simulink model "tank_phase1"  (R2025b)
settings: Solver=ode45  StartTime=0.0  StopTime=900  RelTol=1e-3
model workspace (MAT data in the model file):
  pumpProfile = timeseries
  pumpProfile.Name = 'unnamed'
  pumpProfile.DataInfo = tsdata.datametadata
  pumpProfile.DataInfo.Interpolation = tsdata.interpolation
  pumpProfile.DataInfo.Interpolation.Fhandle : function handle (value not decoded)
  pumpProfile.DataInfo.Interpolation.Name = 'linear'
  pumpProfile.TimeInfo = tsdata.timemetadata
  pumpProfile.TimeInfo.Length = 3
  pumpProfile.TimeInfo.DuplicateTimes = 0
  pumpProfile.TimeInfo.Time_ = [0; 300; 600]
  pumpProfile.TimeInfo.Initialized = 1
  pumpProfile.QualityInfo = tsdata.qualmetadata
  pumpProfile.Data_ = [20; 40; 60]
settings Model: Creator=maild  LastModifiedBy=maild

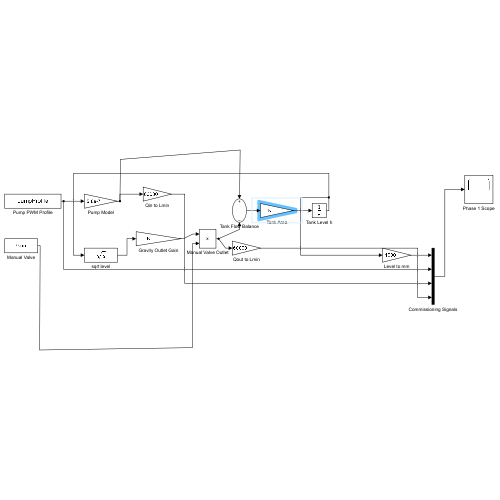
[thumbnail: Simulink's stored preview of the top-level diagram]
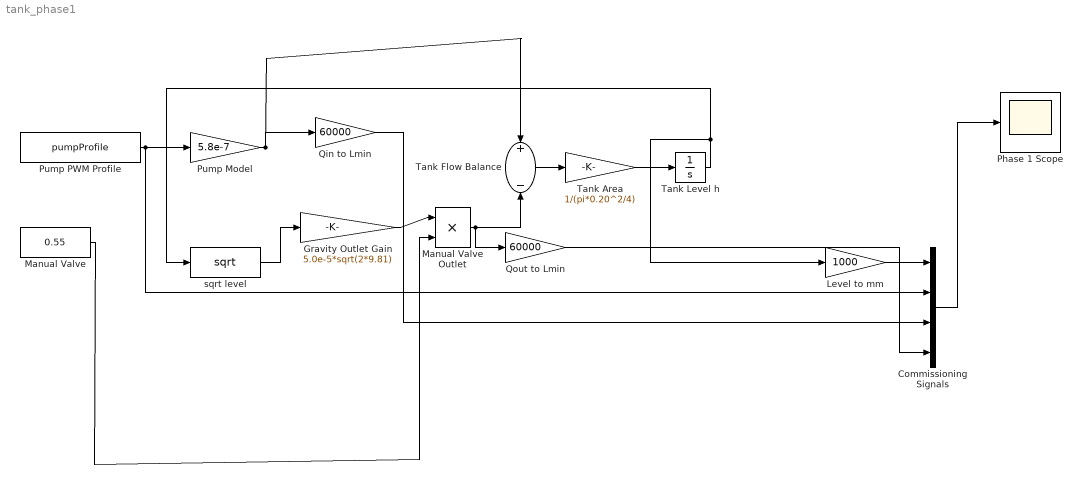
== system tank_phase1 ==
  Commissioning Signals : Mux
  Gravity Outlet Gain : Gain  Gain=5.0e-5*sqrt(2*9.81)
  Level to mm : Gain  Gain=1000
  Manual Valve : Constant  Value=0.55
  Manual Valve Outlet : Product
  Phase 1 Scope : Scope
  Pump Model : Gain  Gain=5.8e-7
  Pump PWM Profile : FromWorkspace  VariableName=pumpProfile
  Qin to Lmin : Gain  Gain=60000
  Qout to Lmin : Gain  Gain=60000
  Tank Area : Gain  Gain=1/(pi*0.20^2/4)
  Tank Flow Balance : Sum  Inputs=+-
  Tank Level h : Integrator  InitialCondition=0.08
  sqrt level : Math  Operator=sqrt
  wires:
  Pump PWM Profile/1 -> Pump Model/1, Commissioning Signals/2
  Pump Model/1 -> Tank Flow Balance/1, Qin to Lmin/1
  Tank Level h/1 -> sqrt level/1, Level to mm/1
  sqrt level/1 -> Gravity Outlet Gain/1
  Gravity Outlet Gain/1 -> Manual Valve Outlet/1
  Manual Valve/1 -> Manual Valve Outlet/2
  Manual Valve Outlet/1 -> Tank Flow Balance/2, Qout to Lmin/1
  Tank Flow Balance/1 -> Tank Area/1
  Tank Area/1 -> Tank Level h/1
  Level to mm/1 -> Commissioning Signals/1
  Qin to Lmin/1 -> Commissioning Signals/3
  Qout to Lmin/1 -> Commissioning Signals/4
  Commissioning Signals/1 -> Phase 1 Scope/1
